simulink model "CD2_Library"  (Simulink 6.4)
settings: Solver=FixedStepDiscrete  StartTime=0  StopTime=7200  FixedStep=300  RelTol=1e-3
InitFcn:
  | CD2_init
undefined symbols (not defined in the file or in its folder): CD2_get_substance_count, CD2_get_substances_count, Crain, get_blocks_id, input_c, subs_vect, table, tablestep
(part 2 of 2)

== system CD2_Library/Mix 3 ==
  " 1" : Inport
  " " : Inport  Port=2
  " 2" : Inport  Port=3
  Mix 8 : Subsystem  mask(Mixer){n_comp=n_comp}
      mask prompts: n_comp "Number of pollutants [ - ]"
      mask help:
      | Performes mixing of pollutant fluxes Q1 and Q2 in accordance to their hydraulic load.
      |
      | Function used:
      | CD1_sfun_mixing_QC.m
      mask init: same as CD2_Library/ 1
      mask Display:
      | plot(0,0,100,100);
      | 
      | text(50,50,'Mix','HorizontalAlignment','center');
      | 
      | 
      | port_label('input',1,'Q1');
      | port_label('input',2,'Q2');
      | port_label('output',1,'Qe');
  Mix 9 : Subsystem  mask(Mixer){n_comp=n_comp}
      mask prompts: n_comp "Number of pollutants [ - ]"
      mask help:
      | Performes mixing of pollutant fluxes Q1 and Q2 in accordance to their hydraulic load.
      |
      | Function used:
      | CD1_sfun_mixing_QC.m
      mask init: same as CD2_Library/ 1
      mask Display:
      | plot(0,0,100,100);
      | 
      | text(50,50,'Mix','HorizontalAlignment','center');
      | 
      | 
      | port_label('input',1,'Q1');
      | port_label('input',2,'Q2');
      | port_label('output',1,'Qe');
  " 3" : Outport
  wires:
  Mix 9/1(" 3") -> Mix 8/1(" 1")
  Mix 8/1(" 3") -> " 3"/1
  " 1"/1 -> Mix 9/1(" 1")
  " "/1 -> Mix 9/2(" ")
  " 2"/1 -> Mix 8/2(" ")

== system CD2_Library/Mix2 ==
  " 1" : Inport
  " " : Inport  Port=2
  Mux : Mux  Inputs=[n_comp+1,n_comp+1]
  S-Function : S-Function  FunctionName=CD1_sfun_mixing_QC  Parameters=n_comp,tstep
  " 3" : Outport
  wires:
  " "/1 -> Mux/2
  S-Function/1 -> " 3"/1
  " 1"/1 -> Mux/1
  Mux/1 -> S-Function/1

== system CD2_Library/Musk oM-Q - 01 ==
  Qi : Inport
  Demux : Demux  Outputs=[N+1,N]
  S-Function1 : S-Function  FunctionName=CD1_sfun_Muskingum_oM_Q  Parameters=dt,N,K,X,C0,C1,C2
  Q : Outport
  V : Outport  Port=2
  wires:
  Qi/1 -> S-Function1/1
  Demux/2 -> V/1
  Demux/1 -> Q/1
  S-Function1/1 -> Demux/1

== system CD2_Library/Musk oS-Q - 01 ==
  Qi : Inport
  Demux : Demux  Outputs=2
  S-Function1 : S-Function  FunctionName=CD1_sfun_Muskingum_oS_Q  Parameters=dt, K, X, C0, C1, C2
  Qe : Outport
  V : Outport  Port=2
  wires:
  S-Function1/1 -> Demux/1
  Demux/1 -> Qe/1
  Demux/2 -> V/1
  Qi/1 -> S-Function1/1

== system CD2_Library/Musk sM-QC - 01 ==
  Qi : Inport
  Demux : Demux  Outputs=2
  S-Function1 : S-Function  FunctionName=CD1_sfun_Muskingum_sM_QC  Parameters=dt, K, X, CA, CB, n_comp,N
  Qe : Outport
  V : Outport  Port=2
  wires:
  S-Function1/1 -> Demux/1
  Demux/1 -> Qe/1
  Demux/2 -> V/1
  Qi/1 -> S-Function1/1

== system CD2_Library/Musk sS-QC - 01 ==
  Qi : Inport
  Demux : Demux  Outputs=2
  S-Function1 : S-Function  FunctionName=CD1_sfun_Muskingum_sS_QC  Parameters=dt, K, X, CA, CB, n_comp
  Qe : Outport
  V : Outport  Port=2
  wires:
  S-Function1/1 -> Demux/1
  Demux/1 -> Qe/1
  Demux/2 -> V/1
  Qi/1 -> S-Function1/1

== system CD2_Library/PE ==
  From DWF : Inport
  Constant : Constant  Value=EG  OutDataType=sfix(16)  ConRadixGroup=Use specified scaling  OutScaling=2^0  SampleTime=inf  FramePeriod=inf
  Product : Product  SaturateOnIntegerOverflow=on
  DWF Q,C : Outport
  wires:
  Product/1 -> DWF Q,C/1
  From DWF/1 -> Product/1
  Constant/1 -> Product/2

== system CD2_Library/Pumping Station ==
  In : Inport
  CSO FirstFlush1 : S-Function  FunctionName=CD1_sfun_pump_A  Parameters=Vmax,NP,Qp,Von,Voff,n_comp,tstep
  Demux : Demux  Outputs=[ (n_comp+1) (n_comp+1) (n_comp+1)]
  Qw : Outport
  Qp : Outport  Port=2
  Vi : Outport  Port=3
  wires:
  Demux/3 -> Vi/1
  Demux/2 -> Qp/1
  Demux/1 -> Qw/1
  CSO FirstFlush1/1 -> Demux/1
  In/1 -> CSO FirstFlush1/1

== system CD2_Library/QCMGENERATOR ==
  S-Function : S-Function  FunctionName=CD1_sfun_dwfgenerator  Parameters=tstep,yy,yye
  DWF : Outport
  wires:
  S-Function/1 -> DWF/1

== system CD2_Library/RAINGENERATOR ==
  S-Function : S-Function  FunctionName=CD1_sfun_raingenerator  Parameters=t_step,a,b,c,d
  Output Signal: mm/timestep : Outport
  wires:
  S-Function/1 -> Output Signal: mm/timestep/1

== system CD2_Library/Rainread ==
  rainread : S-Function  FunctionName=CD1_sfun_rainread  Parameters=crep,table,tablestep,tstep
  out_1 : Outport
  wires:
  rainread/1 -> out_1/1

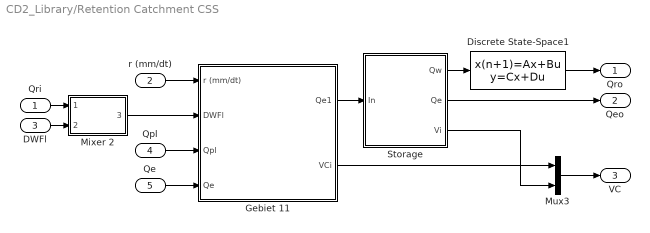
== system CD2_Library/Retention Catchment CSS ==
  Qri : Inport
  r (mm/dt) : Inport  Port=2
  DWFl : Inport  Port=3
  Qpl : Inport  Port=4
  Qe : Inport  Port=5
  " Gebiet 11" : Subsystem  mask(Catchment SSS - Type B){area=area, rfcoeff=rfcoeff, initloss=initloss, permloss=permloss, N=N, n_comp=n_comp, Rain_C=Rain_C, K=K, X=X}
      mask prompts: area "Area in [ha]"; rfcoeff "Runoff coefficient (0 - 1)"; initloss "Initial Loss in [mm]"; permloss "Permanent loss in [mm/day]"; N "No of Timesteps (transport time) / No of subareas n [-]"; n_comp "No of pollutant components"; Rain_C "Vector of Rain-Conc. [g/m3]"
      mask help:
      | Simple model of an urban catchment.
      | Input ( r ) is a continuous stream of rain data in [mm/DT]. Input (DWF) is the dry weather flow. Input (QP) is parasite water flow entering diluting the DWF.
      |
      | Pollutants concentrations for stormwater Qr are considered constant over time. The block contains an initial loss model for runoff generation, a time/area model for overland flow computation and a mixing model for computing runoff concentrations for n components.
      mask init: same as CD2_Library/Catchment CSS
      mask Display:
      | plot(0,0,100,100,
      | [17 20 25 30 40 45 50 55 60 65]+x,
      | [60 80 82 85 88 88 88 85 75 60]+y);
      | plot(0,0,100,100,
      | [17 20 25 30 40 45 50 55 60 65]+x,
      | [55 40 35 30 30 30 30 35 40 55]+y);
      | 
      | plot([20 65]+x,[60 60]+y);
      | plot([20 30]+x,[80 60]+y);
      | plot([30 40]+x,[75 60]+y);
      | plot([45 60]+x,[75 60]+y);
      | plot([20 65]+x,[55 55]+y);
      | plot([20 30]+x,[40 55]+y);
      | plot([30 40]+x,[45 55]+y);
      | plot([45 60]+x,[30 55]+y);
      | 
      | color('black');
      | 
      | port_label('input',1,'rl');
      | port_label('input',2,'DWFl');
      | port_label('input',3,'Qpl');
      | port_label('input',4,'Qe');
      | port_label('output',1,'Qe');
      | port_label('output',2,'VCi');
      | 
      | text(50,90,'CATCHMENT CSS','HorizontalAlignment','center');
  Discrete State-Space1 : DiscreteStateSpace  A=zeros(n_comp+1,n_comp+1)  B=eye(n_comp+1)  C=eye(n_comp+1)  D=zeros(n_comp+1,n_comp+1)  SampleTime=-1
  Mixer 2 : Subsystem  mask(Mixer){n_comp=n_comp}
      mask prompts: n_comp "Number of pollutants [ - ]"
      mask help:
      | Performes mixing of pollutant fluxes Q1 and Q2 in accordance to their hydraulic load.
      |
      | Function used:
      | CD1_sfun_mixing_QC.m
      mask init: same as CD2_Library/ 1
      mask Display:
      | plot(0,0,100,100);
      | 
      | text(50,50,'Mix','HorizontalAlignment','center');
      | 
      | 
      | port_label('input',1,'Q1');
      | port_label('input',2,'Q2');
      | port_label('output',1,'Qe');
  Mux3 : Mux  Inputs=[N*(n_comp+1),n_comp+1]
  Storage : Subsystem  mask(CSO Typ B - Combined sewer overflow){Vmax=Vsmax, Qemax=Qemax, n_comp=n_comp, n_sed=n_sed}
      mask prompts: Vmax "Basin Volume (m3)"; Qemax "Maximum Effluent flow [m3/s]"; n_comp "Number of Pollutants [-]"; n_sed "n-sed (Vect. of Sed. Coefficients)"
      mask help:
      | Combined sewer overflow structure.
      | Diverts the inflow given into effluent and overflow. The model implemented consideres hydraulics and pollutant routing by full mixing in the structure.
      |
      | In addition to Type A a retenetion/sedimentation factor is introduced. The factor may be used for applying different ratios in pollutant concentration for effluent flow (QE) and overflow (QW).
      |
      | Function used:
      | CD1_sfun_cso_B.m
      mask init: same as CD2_Library/ 1
      mask Display:
      | plot(0,0,100,100);
      | 
      | 
      | text(50,60,'CSO','HorizontalAlignment','center');
      | text(50,30,'Typ B','HorizontalAlignment','center');
      | 
      | 
      | port_label('input',1,'Qi');
      | port_label('output',1,'Qw');
      | port_label('output',2,'Qe');
      | port_label('output',3,'Vi');
  Qro : Outport
  Qeo : Outport  Port=2
  VC : Outport  Port=3
  wires:
  Mux3/1 -> VC/1
  Storage/3(Vi) -> Mux3/2
  " Gebiet 11"/2(VCi) -> Mux3/1
  Mixer 2/1(" 3") -> " Gebiet 11"/2(DWFl)
  Qri/1 -> Mixer 2/1(" 1")
  DWFl/1 -> Mixer 2/2(" ")
  Storage/2(Qe) -> Qeo/1
  " Gebiet 11"/1(Qe1) -> Storage/1(In)
  Qe/1 -> " Gebiet 11"/4(Qe)
  Qpl/1 -> " Gebiet 11"/3(Qpl)
  r (mm/dt)/1 -> " Gebiet 11"/1(r (mm/dt))
  Storage/1(Qw) -> Discrete State-Space1/1
  Discrete State-Space1/1 -> Qro/1

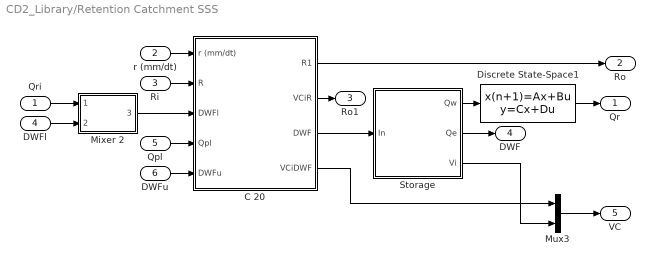
== system CD2_Library/Retention Catchment SSS ==
  Qri : Inport
  r (mm/dt) : Inport  Port=2
  Ri : Inport  Port=3
  DWFl : Inport  Port=4
  Qpl : Inport  Port=5
  DWFu : Inport  Port=6
  " C 20" : Subsystem  mask(Catchment SSS - Type B){area=area, rfcoeff=rfcoeff, initloss=initloss, permloss=permloss, N=N, n_comp=n_comp, Rain_C=Rain_C, K=K, X=X}
      mask prompts: area "Area in [ha]"; rfcoeff "Runoff coefficient (0 - 1)"; initloss "Initial Loss in [mm]"; permloss "Permanent loss in [mm/day]"; N "No of Timesteps (transport time) / No of subareas n [-]"; n_comp "No of pollutant components"; Rain_C "Vector of Rain-Conc. [g/m3]"
      mask help:
      | Simple model of an urban catchment.
      | Input ( r ) is a continuous stream of rain data in [mm/DT]. Input (DWF) is the dry weather flow. Input (QP) is parasite water flow entering diluting the DWF.
      |
      | Pollutants concentrations for stormwater Qr are considered constant over time. The block contains an initial loss model for runoff generation, a time/area model for overland flow computation and a mixing model for computing runoff concentrations for n components.
      mask init: same as CD2_Library/Catchment CSS
      mask Display:
      | plot(0,0,100,100,
      | [17 20 25 30 40 50 55 60 70 75 80]+x,
      | [60 80 82 85 88 88 88 85 82 75 60]+y);
      | 
      | plot([20 80]+x,[60 60]+y);
      | plot([20 30]+x,[80 60]+y);
      | plot([30 40]+x,[75 60]+y);
      | plot([45 60]+x,[75 60]+y);
      | 
      | color('white');
      | plot([20 80]+x,[55 55]+y);
      | plot([20 30]+x,[40 55]+y);
      | plot([30 40]+x,[45 55]+y);
      | plot([45 60]+x,[30 55]+y);
      | 
      | color('black');
      | 
      | port_label('input',1,'rl');
      | port_label('input',2,'R');
      | port_label('input',3,'DWFl');
      | port_label('input',4,'Qpl');
      | port_label('input',5,'DWFu');
      | port_label('output',1,'R');
      | port_label('output',2,'VCi(R)');
      | port_label('output',3,'DWF');
      | port_label('output',4,'VCi(DWF)');
      | 
      | 
      | text(50,90,'CATCHMENT SSS','HorizontalAlignment','center');
  Discrete State-Space1 : DiscreteStateSpace  A=zeros(n_comp+1,n_comp+1)  B=eye(n_comp+1)  C=eye(n_comp+1)  D=zeros(n_comp+1,n_comp+1)  SampleTime=-1
  Mixer 2 : Subsystem  mask(Mixer){n_comp=n_comp}
      mask prompts: n_comp "Number of pollutants [ - ]"
      mask help:
      | Performes mixing of pollutant fluxes Q1 and Q2 in accordance to their hydraulic load.
      |
      | Function used:
      | CD1_sfun_mixing_QC.m
      mask init: same as CD2_Library/ 1
      mask Display:
      | plot(0,0,100,100);
      | 
      | text(50,50,'Mix','HorizontalAlignment','center');
      | 
      | 
      | port_label('input',1,'Q1');
      | port_label('input',2,'Q2');
      | port_label('output',1,'Qe');
  Mux3 : Mux  Inputs=[N*(n_comp+1),n_comp+1]
  Storage : Subsystem  mask(CSO Typ B - Combined sewer overflow){Vmax=Vsmax, Qemax=Qemax, n_comp=n_comp, n_sed=n_sed}
      mask prompts: Vmax "Basin Volume (m3)"; Qemax "Maximum Effluent flow [m3/s]"; n_comp "Number of Pollutants [-]"; n_sed "n-sed (Vect. of Sed. Coefficients)"
      mask help:
      | Combined sewer overflow structure.
      | Diverts the inflow given into effluent and overflow. The model implemented consideres hydraulics and pollutant routing by full mixing in the structure.
      |
      | In addition to Type A a retenetion/sedimentation factor is introduced. The factor may be used for applying different ratios in pollutant concentration for effluent flow (QE) and overflow (QW).
      |
      | Function used:
      | CD1_sfun_cso_B.m
      mask init: same as CD2_Library/ 1
      mask Display:
      | plot(0,0,100,100);
      | 
      | 
      | text(50,60,'CSO','HorizontalAlignment','center');
      | text(50,30,'Typ B','HorizontalAlignment','center');
      | 
      | 
      | port_label('input',1,'Qi');
      | port_label('output',1,'Qw');
      | port_label('output',2,'Qe');
      | port_label('output',3,'Vi');
  Qr : Outport
  Ro : Outport  Port=2
  Ro1 : Outport  Port=3
  "DWF " : Outport  Port=4
  VC : Outport  Port=5
  wires:
  " C 20"/2(VCiR) -> Ro1/1
  Mux3/1 -> VC/1
  Storage/3(Vi) -> Mux3/2
  " C 20"/4(VCiDWF) -> Mux3/1
  DWFl/1 -> Mixer 2/2(" ")
  Qri/1 -> Mixer 2/1(" 1")
  Mixer 2/1(" 3") -> " C 20"/3(DWFl)
  " C 20"/1(R1) -> Ro/1
  " C 20"/3("DWF ") -> Storage/1(In)
  Storage/1(Qw) -> Discrete State-Space1/1
  Storage/2(Qe) -> "DWF "/1
  DWFu/1 -> " C 20"/5(DWFu)
  Qpl/1 -> " C 20"/4(Qpl)
  Ri/1 -> " C 20"/2(R)
  r (mm/dt)/1 -> " C 20"/1(r (mm/dt))
  Discrete State-Space1/1 -> Qr/1

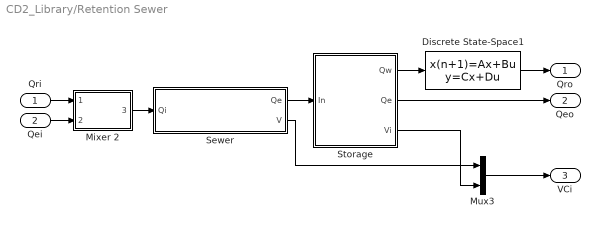
== system CD2_Library/Retention Sewer ==
  Qri : Inport
  Qei : Inport  Port=2
  Discrete State-Space1 : DiscreteStateSpace  A=zeros(n_comp+1,n_comp+1)  B=eye(n_comp+1)  C=eye(n_comp+1)  D=zeros(n_comp+1,n_comp+1)  SampleTime=-1
  Mixer 2 : Subsystem  mask(Mixer){n_comp=n_comp}
      mask prompts: n_comp "Number of pollutants [ - ]"
      mask help:
      | Performes mixing of pollutant fluxes Q1 and Q2 in accordance to their hydraulic load.
      |
      | Function used:
      | CD1_sfun_mixing_QC.m
      mask init: same as CD2_Library/ 1
      mask Display:
      | plot(0,0,100,100);
      | 
      | text(50,50,'Mix','HorizontalAlignment','center');
      | 
      | 
      | port_label('input',1,'Q1');
      | port_label('input',2,'Q2');
      | port_label('output',1,'Qe');
  Mux3 : Mux  Inputs=[N*(n_comp+1),n_comp+1]
  Sewer : Subsystem  mask(Muskingum simplified scheme for Sewer){K=K, X=X, n_comp=n_comp, N=N}
      mask prompts: K "K (travel time of a subreach) [s]"; X "X (weighing factor)  [ - ]"; n_comp "Number of pollutants [ - ]"; N "N (Number of sub-reaches) [ - ]"
      mask help:
      | Function used:
      | CD1_sfun_Muskingum_Sewer.m
      mask init: same as CD2_Library/Sewer
      mask Display:
      | plot(0,0,100,50,
      | [0,50,50,0,0]+x,[-10,-10,10,10,-10]+y,
      | [10,10]+x,[-10,10]+y,
      | [20,20]+x,[-10,10]+y,
      | [30,30]+x,[-10,10]+y,
      | [40,40]+x,[-10,10]+y,
      | [0,0,5,5,10,5,5,0]+kx,
      | [5,-5,-5,-13,0,13,5,5]+ky
      | );
      | 
      | 
      | text(50,7,'SEWER sM','HorizontalAlignment','center');
      | 
      | port_label('input',1,'Qi');
      | port_label('output',1,'Qe');
      | port_label('output',2,'VCi');
  Storage : Subsystem  mask(CSO Typ B - Combined sewer overflow){Vmax=Vsmax, Qemax=Qemax, n_comp=n_comp, n_sed=n_sed}
      mask prompts: Vmax "Basin Volume (m3)"; Qemax "Maximum Effluent flow [m3/s]"; n_comp "Number of Pollutants [-]"; n_sed "n-sed (Vect. of Sed. Coefficients)"
      mask help:
      | Combined sewer overflow structure.
      | Diverts the inflow given into effluent and overflow. The model implemented consideres hydraulics and pollutant routing by full mixing in the structure.
      |
      | In addition to Type A a retenetion/sedimentation factor is introduced. The factor may be used for applying different ratios in pollutant concentration for effluent flow (QE) and overflow (QW).
      |
      | Function used:
      | CD1_sfun_cso_B.m
      mask init: same as CD2_Library/ 1
      mask Display:
      | plot(0,0,100,100);
      | 
      | 
      | text(50,60,'CSO','HorizontalAlignment','center');
      | text(50,30,'Typ B','HorizontalAlignment','center');
      | 
      | 
      | port_label('input',1,'Qi');
      | port_label('output',1,'Qw');
      | port_label('output',2,'Qe');
      | port_label('output',3,'Vi');
  Qro : Outport
  Qeo : Outport  Port=2
  VCi : Outport  Port=3
  wires:
  Storage/3(Vi) -> Mux3/2
  Sewer/2(V) -> Mux3/1
  Sewer/1(Qe) -> Storage/1(In)
  Mixer 2/1(" 3") -> Sewer/1(Qi)
  Storage/2(Qe) -> Qeo/1
  Qri/1 -> Mixer 2/1(" 1")
  Qei/1 -> Mixer 2/2(" ")
  Mux3/1 -> VCi/1
  Storage/1(Qw) -> Discrete State-Space1/1
  Discrete State-Space1/1 -> Qro/1

== system CD2_Library/Set Substance ==
  " 1" : Inport
  " " : Inport  Port=2
  Mux : Mux  Inputs=[CD2_get_substance_count(subs_vect),n_comp+1]
  S-Function : S-Function  FunctionName=CD2_sfun_mixing_QC_subs  Parameters=subs_vect,n_comp,tstep
  " 3" : Outport
  wires:
  Mux/1 -> S-Function/1
  " 1"/1 -> Mux/1
  S-Function/1 -> " 3"/1
  " "/1 -> Mux/2

== system CD2_Library/SetGlobalVariable ==

== system CD2_Library/Sewer ==
  Qi : Inport
  Demux : Demux  Outputs=[n_comp+1,N*(n_comp+1)]
  S-Function1 : S-Function  FunctionName=CD1_sfun_Muskingum_Sewer  Parameters=dt, K, X, CA, CB, n_comp,N
  Qe : Outport
  V : Outport  Port=2
  wires:
  Qi/1 -> S-Function1/1
  Demux/2 -> V/1
  Demux/1 -> Qe/1
  S-Function1/1 -> Demux/1

== system CD2_Library/Splitter  ==
  " 1" : Inport
  Demux : Demux  Outputs=2
  S-Function : S-Function  FunctionName=CD1_sfun_splitter  Parameters=n_comp,values,mode,tstep
  " 3" : Outport
  " 2" : Outport  Port=2
  wires:
  " 1"/1 -> S-Function/1  "inpt"
  S-Function/1 -> Demux/1
  Demux/1 -> " 3"/1
  Demux/2 -> " 2"/1

== system CD2_Library/Substance Filter ==
  " 1" : Inport
  S-Function : S-Function  FunctionName=CD2_sfun_out_subs  Parameters=subs_vect,n_comp,tstep
  " 3" : Outport
  wires:
  S-Function/1 -> " 3"/1
  " 1"/1 -> S-Function/1

== system CD2_Library/Switcher ==
  " 1" : Inport
  " " : Inport  Port=2
  Mux : Mux  Inputs=[n_comp+1,n_comp+1]
  S-Function : S-Function  FunctionName=CD1_sfun_switcher  Parameters=wechsler,n_comp,tstep
  " 3" : Outport
  wires:
  " 1"/1 -> Mux/1
  " "/1 -> Mux/2
  Mux/1 -> S-Function/1
  S-Function/1 -> " 3"/1

== system CD2_Library/WWTP ==
  In : Inport
  WWTP v01 - 1 : S-Function  FunctionName=CD1_sfun_WWTP  Parameters=n_comp,RE,Cemax,tstep
  Qw : Outport
  wires:
  In/1 -> WWTP v01 - 1/1
  WWTP v01 - 1/1 -> Qw/1

== system CD2_Library/Mix 3/Mix 8 ==
  " 1" : Inport
  " " : Inport  Port=2
  Mux : Mux  Inputs=[n_comp+1,n_comp+1]
  S-Function : S-Function  FunctionName=CD1_sfun_mixing_QC  Parameters=n_comp,tstep
  " 3" : Outport
  wires:
  Mux/1 -> S-Function/1
  " 1"/1 -> Mux/1
  S-Function/1 -> " 3"/1
  " "/1 -> Mux/2

== system CD2_Library/Mix 3/Mix 9 ==
  " 1" : Inport
  " " : Inport  Port=2
  Mux : Mux  Inputs=[n_comp+1,n_comp+1]
  S-Function : S-Function  FunctionName=CD1_sfun_mixing_QC  Parameters=n_comp,tstep
  " 3" : Outport
  wires:
  Mux/1 -> S-Function/1
  " 1"/1 -> Mux/1
  S-Function/1 -> " 3"/1
  " "/1 -> Mux/2

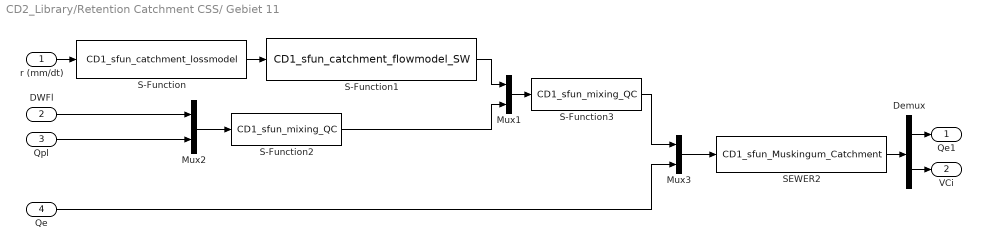
== system CD2_Library/Retention Catchment CSS/ Gebiet 11 ==
  r (mm/dt) : Inport
  DWFl : Inport  Port=2
  Qpl : Inport  Port=3
  Qe : Inport  Port=4
  Demux : Demux  Outputs=[n_comp+1,N*(n_comp+1)]
  Mux1 : Mux  Inputs=[n_comp+1,n_comp+1]
  Mux2 : Mux  Inputs=[n_comp+1,n_comp+1]
  Mux3 : Mux  Inputs=[n_comp+1,n_comp+1]
  S-Function : S-Function  FunctionName=CD1_sfun_catchment_lossmodel  Parameters=initloss,permloss,rfcoeff
  S-Function1 : S-Function  FunctionName=CD1_sfun_catchment_flowmodel_SW  Parameters=area,n_comp,Rain_C,tstep
  S-Function2 : S-Function  FunctionName=CD1_sfun_mixing_QC  Parameters=n_comp,tstep
  S-Function3 : S-Function  FunctionName=CD1_sfun_mixing_QC  Parameters=n_comp,tstep
  SEWER2 : S-Function  FunctionName=CD1_sfun_Muskingum_Catchment  Parameters=tstep, CX, CY, n_comp,N
  Qe1 : Outport
  VCi : Outport  Port=2
  wires:
  S-Function1/1 -> Mux1/1
  Mux2/1 -> S-Function2/1
  r (mm/dt)/1 -> S-Function/1
  S-Function/1 -> S-Function1/1
  Qpl/1 -> Mux2/2
  DWFl/1 -> Mux2/1
  S-Function2/1 -> Mux1/2
  Mux1/1 -> S-Function3/1
  S-Function3/1 -> Mux3/1
  Qe/1 -> Mux3/2
  Mux3/1 -> SEWER2/1
  SEWER2/1 -> Demux/1
  Demux/1 -> Qe1/1
  Demux/2 -> VCi/1

== system CD2_Library/Retention Catchment CSS/Mixer 2 ==
  " 1" : Inport
  " " : Inport  Port=2
  Mux : Mux  Inputs=[n_comp+1,n_comp+1]
  S-Function : S-Function  FunctionName=CD1_sfun_mixing_QC  Parameters=n_comp,tstep
  " 3" : Outport
  wires:
  " "/1 -> Mux/2
  S-Function/1 -> " 3"/1
  " 1"/1 -> Mux/1
  Mux/1 -> S-Function/1

== system CD2_Library/Retention Catchment CSS/Storage ==
  In : Inport
  Catchment Storage : S-Function  FunctionName=CD1_sfun_cso_B  Parameters=Vmax,Qemax,n_comp,n_sed,tstep
  Demux : Demux  Outputs=[ (n_comp+1) (n_comp+1) (n_comp+1)]
  Qw : Outport
  Qe : Outport  Port=2
  Vi : Outport  Port=3
  wires:
  In/1 -> Catchment Storage/1
  Catchment Storage/1 -> Demux/1
  Demux/1 -> Qw/1
  Demux/2 -> Qe/1
  Demux/3 -> Vi/1

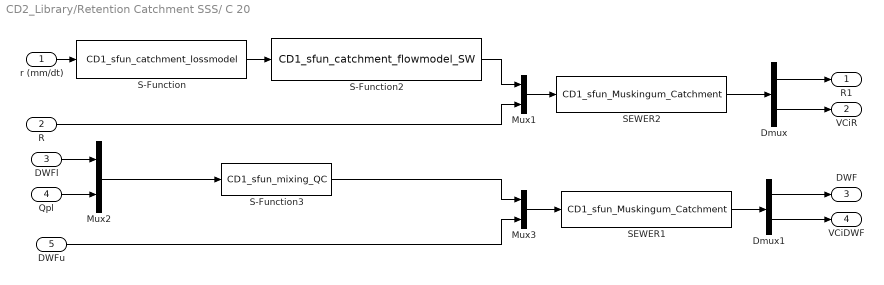
== system CD2_Library/Retention Catchment SSS/ C 20 ==
  r (mm/dt) : Inport
  R : Inport  Port=2
  DWFl : Inport  Port=3
  Qpl : Inport  Port=4
  DWFu : Inport  Port=5
  Dmux : Demux  Outputs=[n_comp+1,N*(n_comp+1)]
  Dmux1 : Demux  Outputs=[n_comp+1,N*(n_comp+1)]
  Mux1 : Mux  Inputs=[n_comp+1,n_comp+1]
  Mux2 : Mux  Inputs=[n_comp+1,n_comp+1]
  Mux3 : Mux  Inputs=[n_comp+1,n_comp+1]
  S-Function : S-Function  FunctionName=CD1_sfun_catchment_lossmodel  Parameters=initloss,permloss,rfcoeff
  S-Function2 : S-Function  FunctionName=CD1_sfun_catchment_flowmodel_SW  Parameters=area,n_comp,Rain_C,tstep
  S-Function3 : S-Function  FunctionName=CD1_sfun_mixing_QC  Parameters=n_comp,tstep
  SEWER1 : S-Function  FunctionName=CD1_sfun_Muskingum_Catchment  Parameters=tstep, CX, CY, n_comp,N
  SEWER2 : S-Function  FunctionName=CD1_sfun_Muskingum_Catchment  Parameters=tstep, CX, CY, n_comp,N
  R1 : Outport
  VCiR : Outport  Port=2
  "DWF " : Outport  Port=3
  VCiDWF : Outport  Port=4
  wires:
  S-Function/1 -> S-Function2/1
  r (mm/dt)/1 -> S-Function/1
  DWFl/1 -> Mux2/1
  R/1 -> Mux1/2
  S-Function2/1 -> Mux1/1
  Mux1/1 -> SEWER2/1
  Mux3/1 -> SEWER1/1
  SEWER2/1 -> Dmux/1
  Dmux/1 -> R1/1
  SEWER1/1 -> Dmux1/1
  Dmux1/1 -> "DWF "/1
  Dmux/2 -> VCiR/1
  Dmux1/2 -> VCiDWF/1
  Qpl/1 -> Mux2/2
  Mux2/1 -> S-Function3/1
  S-Function3/1 -> Mux3/1
  DWFu/1 -> Mux3/2

== system CD2_Library/Retention Catchment SSS/Mixer 2 ==
  " 1" : Inport
  " " : Inport  Port=2
  Mux : Mux  Inputs=[n_comp+1,n_comp+1]
  S-Function : S-Function  FunctionName=CD1_sfun_mixing_QC  Parameters=n_comp,tstep
  " 3" : Outport
  wires:
  " "/1 -> Mux/2
  S-Function/1 -> " 3"/1
  " 1"/1 -> Mux/1
  Mux/1 -> S-Function/1

== system CD2_Library/Retention Catchment SSS/Storage ==
  In : Inport
  CSO FirstFlush1 : S-Function  FunctionName=CD1_sfun_cso_B  Parameters=Vmax,Qemax,n_comp,n_sed,tstep
  Demux : Demux  Outputs=[ (n_comp+1) (n_comp+1) (n_comp+1)]
  Qw : Outport
  Qe : Outport  Port=2
  Vi : Outport  Port=3
  wires:
  In/1 -> CSO FirstFlush1/1
  CSO FirstFlush1/1 -> Demux/1
  Demux/1 -> Qw/1
  Demux/2 -> Qe/1
  Demux/3 -> Vi/1

== system CD2_Library/Retention Sewer/Mixer 2 ==
  " 1" : Inport
  " " : Inport  Port=2
  Mux : Mux  Inputs=[n_comp+1,n_comp+1]
  S-Function : S-Function  FunctionName=CD1_sfun_mixing_QC  Parameters=n_comp,tstep
  " 3" : Outport
  wires:
  Mux/1 -> S-Function/1
  " 1"/1 -> Mux/1
  S-Function/1 -> " 3"/1
  " "/1 -> Mux/2

== system CD2_Library/Retention Sewer/Sewer ==
  Qi : Inport
  Demux : Demux  Outputs=[n_comp+1,N*(n_comp+1)]
  S-Function1 : S-Function  FunctionName=CD1_sfun_Muskingum_Sewer  Parameters=dt, K, X, CA, CB, n_comp,N
  Qe : Outport
  V : Outport  Port=2
  wires:
  Qi/1 -> S-Function1/1
  Demux/2 -> V/1
  Demux/1 -> Qe/1
  S-Function1/1 -> Demux/1

== system CD2_Library/Retention Sewer/Storage ==
  In : Inport
  CSO FirstFlush1 : S-Function  FunctionName=CD1_sfun_cso_B  Parameters=Vmax,Qemax,n_comp,n_sed,tstep
  Demux : Demux  Outputs=[ (n_comp+1) (n_comp+1) (n_comp+1)]
  Qw : Outport
  Qe : Outport  Port=2
  Vi : Outport  Port=3
  wires:
  Demux/3 -> Vi/1
  Demux/2 -> Qe/1
  Demux/1 -> Qw/1
  CSO FirstFlush1/1 -> Demux/1
  In/1 -> CSO FirstFlush1/1
